simulink model "SPwm_FOC_5phase"  (R2024b)
settings: Solver=VariableStepAuto  StartTime=0.0  StopTime=0.5  RelTol=1e-3
InitFcn:
  | Pn=4;
  | Ts=5e-7;
  | Tsample=1e-4;
  | Ld=1.35e-3;
  | Lq=1.35e-3;
  | R=2.875;
  | flux=0.05;
  | J=0.002;
  | B=0.02;
  | fc=500;
libraries: spsIGBTDiodeLib x10, spsVIMeasurementModel x7, spsCurrentMeasurementLib x5, spsVoltageMeasurementLib x5, slpidlib x5, spsGroundLib x2, spsDCVoltageSourceLib x1, spsPermanentMagnetSynchronousMachineLib x1, sps_lib x1, simulink x1
settings Model: Creator=23954  LastModifiedBy=23954

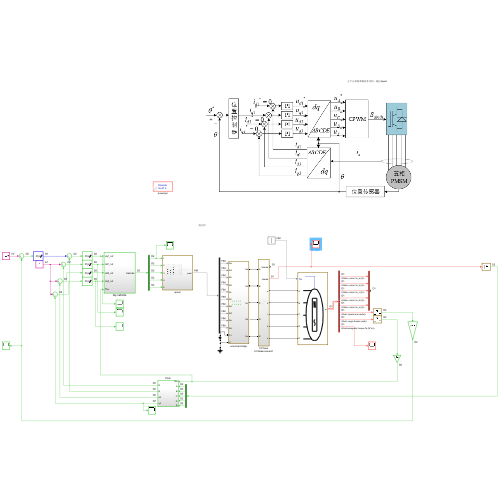
[thumbnail: Simulink's stored preview of the top-level diagram]
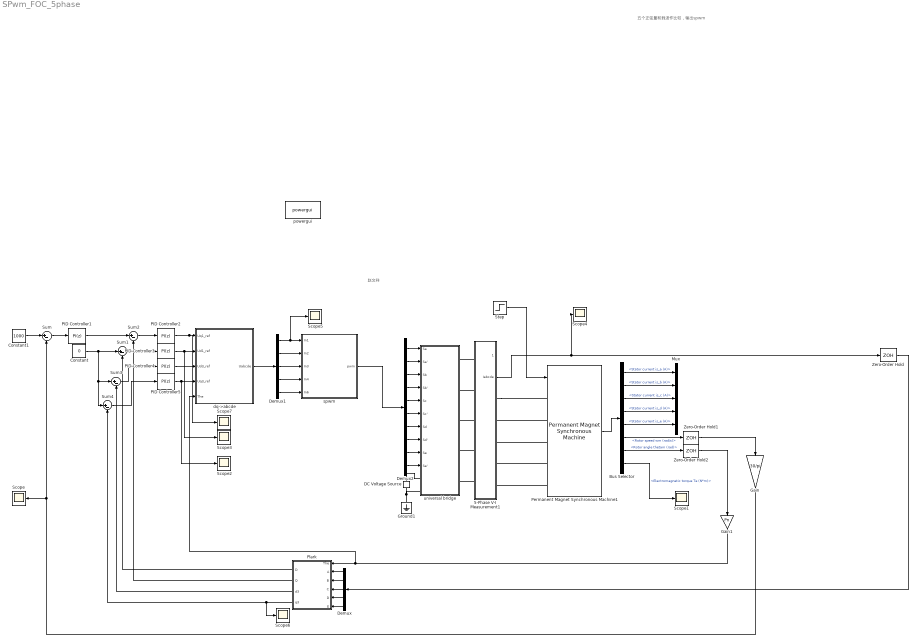
== system SPwm_FOC_5phase ==
  note: 赵文祥
  note: 五个正弦量和载波作比较，输出spwm
  5-Phase V-I Measurement1 : Subsystem
  Bus Selector : BusSelector  OutputSignals=Stator current is_a (A),Stator current is_b (A),Stator current is_c (A),Stator current is_d (A),Stator current is_e (A),Rotor speed wm (rad/s),Rotor angle thetam (rad),Electromagnetic torque Te (N*m)
  Constant : Constant  Value=0
  Constant1 : Constant  Value=1000
  DC Voltage Source : spsDCVoltageSourceLib/DC Voltage Source  Amplitude=311  Measurements=None
  Demux : Demux  Outputs=5
  Demux1 : Demux  Outputs=5
  Demux2 : Demux  Outputs=10
  Gain : Gain  Gain=30/pi
  Gain1 : Gain  Gain=Pn
  Ground1 : spsGroundLib/Ground  LConnTagsString=a
  Mux : Mux  Inputs=5
  PID Controller1 : slpidlib/PID Controller  Controller=PI  Form=Parallel  TimeDomain=Discrete-time  UseExternalTs=off  SampleTime=1e-3  IntegratorMethod=Forward Euler  FilterMethod=Forward Euler  ControllerParametersSource=internal  P=0.02  I=0.02*20  UseKiTs=off  D=0  UseExternalDerivativeSource=off  N=100  UseFilter=on  TunerSelectOption=Transfer Function Based (PID Tuner App)  InitialConditionSource=internal  InitialConditionForIntegrator=0  InitialConditionForFilter=0  DifferentiatorICPrevScaledInput=0  ExternalReset=none  TrackingMode=off  Kt=1  LimitOutput=on  SatLimitsSource=internal  UpperSaturationLimit=150  LowerSaturationLimit=-150  LinearizeAsGain=on  AntiWindupMode=none  Kb=1  LimitIntegrator=off  UpperIntegratorSaturationLimit=inf  LowerIntegratorSaturationLimit=-inf  POutMin=[]  POutMax=[]  IOutMin=[]  IOutMax=[]  DOutMin=[]  DOutMax=[]  NOutMin=[]  NOutMax=[]  SumOutMin=[]  SumOutMax=[]  SaturationOutMin=[]  SaturationOutMax=[]  PParamMin=[]  PParamMax=[]  IParamMin=[]  IParamMax=[]  DParamMin=[]  DParamMax=[]  NParamMin=[]  NParamMax=[]  KbParamMin=[]  KbParamMax=[]  KtParamMin=[]  KtParamMax=[]  KbOutMin=[]  KbOutMax=[]  KtOutMin=[]  KtOutMax=[]  IntegratorOutMin=[]  IntegratorOutMax=[]  FilterOutMin=[]  FilterOutMax=[]  SumI1OutMin=[]  SumI1OutMax=[]  SumI2OutMin=[]  SumI2OutMax=[]  SumI3OutMin=[]  SumI3OutMax=[]  SumI4OutMin=[]  SumI4OutMax=[]  SumDOutMin=[]  SumDOutMax=[]  DifferentiatorOutMin=[]  DifferentiatorOutMax=[]  FilterDiffOutCoefMin=[]  FilterDiffOutCoefMax=[]  ReciprocalOutMin=[]  ReciprocalOutMax=[]  SumDenOutMin=[]  SumDenOutMax=[]  SumNumOutMin=[]  SumNumOutMax=[]  DivideOutMin=[]  DivideOutMax=[]  UdiffTsProdOutMin=[]  UdiffTsProdOutMax=[]  NTsProdOutMin=[]  NTsProdOutMax=[]  UintegralTsProdOutMin=[]  UintegralTsProdOutMax=[]  UngainTsProdOutMin=[]  UngainTsProdOutMax=[]  ClampingZeroOutDataTypeStr=Inherit: Inherit via back propagation  ClampingZeroOutMin=[]  ClampingZeroOutMax=[]  FilterDenConstantOutDataTypeStr=Inherit: Inherit via back propagation  FilterDenConstantOutMin=[]  FilterDenConstantOutMax=[]  PCopyOutDataTypeStr=Inherit: Inherit via back propagation  PCopyOutMin=[]  PCopyOutMax=[]  NCopyOutDataTypeStr=Inherit: Inherit via back propagation  NCopyOutMin=[]  NCopyOutMax=[]  IntegratorContinuousStateAttributes=''  IntegratorStateMustResolveToSignalObject=off  IntegratorRTWStateStorageClass=Auto  FilterContinuousStateAttributes=''  FilterStateMustResolveToSignalObject=off  FilterRTWStateStorageClass=Auto  ParallelPVariant=InternalParameters  IdealPVariant=Disabled  IVariant=InternalParameters  DVariant=Disabled  IntegratorVariant=Discrete  SatVariant=Enabled  AWVariant=Passthrough  PCopyVariant=Disabled  TRVariant=Disabled  FdbkBlocksVariant=Forward  IdealPFdbkVariant=Disabled  SatFdbkVariant=Disabled  DerivativeFilterVariant=Disabled  NVariant=Disabled  NCopyVariant=Disabled_SignalSpec  FilterICVariant=Disabled  IntegratorICVariant=InternalICs  ExternalResetVariant=Disabled  TRSumVariant=Passthrough  SumFdbkVariant=Disabled  SumVariant=Sum_PI  TsampFilterVariant=InternalTs  TsampNgainVariant=Passthrough  TsampIntegralVariant=Disabled_SignalSpec  ExternalSaturationOutDataTypeStr=Inherit: Same as second input  DerivativeSourceVariant=Disabled  PreIntVariant=InternalPreInt
  PID Controller2 : slpidlib/PID Controller  Controller=PI  Form=Parallel  TimeDomain=Discrete-time  UseExternalTs=off  SampleTime=Tsample  IntegratorMethod=Forward Euler  FilterMethod=Forward Euler  ControllerParametersSource=internal  P=Lq*1000  I=R*1100  UseKiTs=off  D=0  UseExternalDerivativeSource=off  N=100  UseFilter=on  TunerSelectOption=Transfer Function Based (PID Tuner App)  InitialConditionSource=internal  InitialConditionForIntegrator=0  InitialConditionForFilter=0  DifferentiatorICPrevScaledInput=0  ExternalReset=none  TrackingMode=off  Kt=1  LimitOutput=on  SatLimitsSource=internal  UpperSaturationLimit=150  LowerSaturationLimit=-150  LinearizeAsGain=on  AntiWindupMode=none  Kb=1  LimitIntegrator=off  UpperIntegratorSaturationLimit=inf  LowerIntegratorSaturationLimit=-inf  POutMin=[]  POutMax=[]  IOutMin=[]  IOutMax=[]  DOutMin=[]  DOutMax=[]  NOutMin=[]  NOutMax=[]  SumOutMin=[]  SumOutMax=[]  SaturationOutMin=[]  SaturationOutMax=[]  PParamMin=[]  PParamMax=[]  IParamMin=[]  IParamMax=[]  DParamMin=[]  DParamMax=[]  NParamMin=[]  NParamMax=[]  KbParamMin=[]  KbParamMax=[]  KtParamMin=[]  KtParamMax=[]  KbOutMin=[]  KbOutMax=[]  KtOutMin=[]  KtOutMax=[]  IntegratorOutMin=[]  IntegratorOutMax=[]  FilterOutMin=[]  FilterOutMax=[]  SumI1OutMin=[]  SumI1OutMax=[]  SumI2OutMin=[]  SumI2OutMax=[]  SumI3OutMin=[]  SumI3OutMax=[]  SumI4OutMin=[]  SumI4OutMax=[]  SumDOutMin=[]  SumDOutMax=[]  DifferentiatorOutMin=[]  DifferentiatorOutMax=[]  FilterDiffOutCoefMin=[]  FilterDiffOutCoefMax=[]  ReciprocalOutMin=[]  ReciprocalOutMax=[]  SumDenOutMin=[]  SumDenOutMax=[]  SumNumOutMin=[]  SumNumOutMax=[]  DivideOutMin=[]  DivideOutMax=[]  UdiffTsProdOutMin=[]  UdiffTsProdOutMax=[]  NTsProdOutMin=[]  NTsProdOutMax=[]  UintegralTsProdOutMin=[]  UintegralTsProdOutMax=[]  UngainTsProdOutMin=[]  UngainTsProdOutMax=[]  ClampingZeroOutDataTypeStr=Inherit: Inherit via back propagation  ClampingZeroOutMin=[]  ClampingZeroOutMax=[]  FilterDenConstantOutDataTypeStr=Inherit: Inherit via back propagation  FilterDenConstantOutMin=[]  FilterDenConstantOutMax=[]  PCopyOutDataTypeStr=Inherit: Inherit via back propagation  PCopyOutMin=[]  PCopyOutMax=[]  NCopyOutDataTypeStr=Inherit: Inherit via back propagation  NCopyOutMin=[]  NCopyOutMax=[]  IntegratorContinuousStateAttributes=''  IntegratorStateMustResolveToSignalObject=off  IntegratorRTWStateStorageClass=Auto  FilterContinuousStateAttributes=''  FilterStateMustResolveToSignalObject=off  FilterRTWStateStorageClass=Auto  ParallelPVariant=InternalParameters  IdealPVariant=Disabled  IVariant=InternalParameters  DVariant=Disabled  IntegratorVariant=Discrete  SatVariant=Enabled  AWVariant=Passthrough  PCopyVariant=Disabled  TRVariant=Disabled  FdbkBlocksVariant=Forward  IdealPFdbkVariant=Disabled  SatFdbkVariant=Disabled  DerivativeFilterVariant=Disabled  NVariant=Disabled  NCopyVariant=Disabled_SignalSpec  FilterICVariant=Disabled  IntegratorICVariant=InternalICs  ExternalResetVariant=Disabled  TRSumVariant=Passthrough  SumFdbkVariant=Disabled  SumVariant=Sum_PI  TsampFilterVariant=InternalTs  TsampNgainVariant=Passthrough  TsampIntegralVariant=Disabled_SignalSpec  ExternalSaturationOutDataTypeStr=Inherit: Same as second input  DerivativeSourceVariant=Disabled  PreIntVariant=InternalPreInt
  PID Controller3 : slpidlib/PID Controller  Controller=PI  Form=Parallel  TimeDomain=Discrete-time  UseExternalTs=off  SampleTime=Tsample  IntegratorMethod=Forward Euler  FilterMethod=Forward Euler  ControllerParametersSource=internal  P=Ld*1000  I=R*1100  UseKiTs=off  D=0  UseExternalDerivativeSource=off  N=100  UseFilter=on  TunerSelectOption=Transfer Function Based (PID Tuner App)  InitialConditionSource=internal  InitialConditionForIntegrator=0  InitialConditionForFilter=0  DifferentiatorICPrevScaledInput=0  ExternalReset=none  TrackingMode=off  Kt=1  LimitOutput=on  SatLimitsSource=internal  UpperSaturationLimit=150  LowerSaturationLimit=-150  LinearizeAsGain=on  AntiWindupMode=none  Kb=1  LimitIntegrator=off  UpperIntegratorSaturationLimit=inf  LowerIntegratorSaturationLimit=-inf  POutMin=[]  POutMax=[]  IOutMin=[]  IOutMax=[]  DOutMin=[]  DOutMax=[]  NOutMin=[]  NOutMax=[]  SumOutMin=[]  SumOutMax=[]  SaturationOutMin=[]  SaturationOutMax=[]  PParamMin=[]  PParamMax=[]  IParamMin=[]  IParamMax=[]  DParamMin=[]  DParamMax=[]  NParamMin=[]  NParamMax=[]  KbParamMin=[]  KbParamMax=[]  KtParamMin=[]  KtParamMax=[]  KbOutMin=[]  KbOutMax=[]  KtOutMin=[]  KtOutMax=[]  IntegratorOutMin=[]  IntegratorOutMax=[]  FilterOutMin=[]  FilterOutMax=[]  SumI1OutMin=[]  SumI1OutMax=[]  SumI2OutMin=[]  SumI2OutMax=[]  SumI3OutMin=[]  SumI3OutMax=[]  SumI4OutMin=[]  SumI4OutMax=[]  SumDOutMin=[]  SumDOutMax=[]  DifferentiatorOutMin=[]  DifferentiatorOutMax=[]  FilterDiffOutCoefMin=[]  FilterDiffOutCoefMax=[]  ReciprocalOutMin=[]  ReciprocalOutMax=[]  SumDenOutMin=[]  SumDenOutMax=[]  SumNumOutMin=[]  SumNumOutMax=[]  DivideOutMin=[]  DivideOutMax=[]  UdiffTsProdOutMin=[]  UdiffTsProdOutMax=[]  NTsProdOutMin=[]  NTsProdOutMax=[]  UintegralTsProdOutMin=[]  UintegralTsProdOutMax=[]  UngainTsProdOutMin=[]  UngainTsProdOutMax=[]  ClampingZeroOutDataTypeStr=Inherit: Inherit via back propagation  ClampingZeroOutMin=[]  ClampingZeroOutMax=[]  FilterDenConstantOutDataTypeStr=Inherit: Inherit via back propagation  FilterDenConstantOutMin=[]  FilterDenConstantOutMax=[]  PCopyOutDataTypeStr=Inherit: Inherit via back propagation  PCopyOutMin=[]  PCopyOutMax=[]  NCopyOutDataTypeStr=Inherit: Inherit via back propagation  NCopyOutMin=[]  NCopyOutMax=[]  IntegratorContinuousStateAttributes=''  IntegratorStateMustResolveToSignalObject=off  IntegratorRTWStateStorageClass=Auto  FilterContinuousStateAttributes=''  FilterStateMustResolveToSignalObject=off  FilterRTWStateStorageClass=Auto  ParallelPVariant=InternalParameters  IdealPVariant=Disabled  IVariant=InternalParameters  DVariant=Disabled  IntegratorVariant=Discrete  SatVariant=Enabled  AWVariant=Passthrough  PCopyVariant=Disabled  TRVariant=Disabled  FdbkBlocksVariant=Forward  IdealPFdbkVariant=Disabled  SatFdbkVariant=Disabled  DerivativeFilterVariant=Disabled  NVariant=Disabled  NCopyVariant=Disabled_SignalSpec  FilterICVariant=Disabled  IntegratorICVariant=InternalICs  ExternalResetVariant=Disabled  TRSumVariant=Passthrough  SumFdbkVariant=Disabled  SumVariant=Sum_PI  TsampFilterVariant=InternalTs  TsampNgainVariant=Passthrough  TsampIntegralVariant=Disabled_SignalSpec  ExternalSaturationOutDataTypeStr=Inherit: Same as second input  DerivativeSourceVariant=Disabled  PreIntVariant=InternalPreInt
  PID Controller4 : slpidlib/PID Controller  Controller=PI  Form=Parallel  TimeDomain=Discrete-time  UseExternalTs=off  SampleTime=Tsample  IntegratorMethod=Forward Euler  FilterMethod=Forward Euler  ControllerParametersSource=internal  P=Ld*1000  I=R*1100  UseKiTs=off  D=0  UseExternalDerivativeSource=off  N=100  UseFilter=on  TunerSelectOption=Transfer Function Based (PID Tuner App)  InitialConditionSource=internal  InitialConditionForIntegrator=0  InitialConditionForFilter=0  DifferentiatorICPrevScaledInput=0  ExternalReset=none  TrackingMode=off  Kt=1  LimitOutput=on  SatLimitsSource=internal  UpperSaturationLimit=150  LowerSaturationLimit=-150  LinearizeAsGain=on  AntiWindupMode=none  Kb=1  LimitIntegrator=off  UpperIntegratorSaturationLimit=inf  LowerIntegratorSaturationLimit=-inf  POutMin=[]  POutMax=[]  IOutMin=[]  IOutMax=[]  DOutMin=[]  DOutMax=[]  NOutMin=[]  NOutMax=[]  SumOutMin=[]  SumOutMax=[]  SaturationOutMin=[]  SaturationOutMax=[]  PParamMin=[]  PParamMax=[]  IParamMin=[]  IParamMax=[]  DParamMin=[]  DParamMax=[]  NParamMin=[]  NParamMax=[]  KbParamMin=[]  KbParamMax=[]  KtParamMin=[]  KtParamMax=[]  KbOutMin=[]  KbOutMax=[]  KtOutMin=[]  KtOutMax=[]  IntegratorOutMin=[]  IntegratorOutMax=[]  FilterOutMin=[]  FilterOutMax=[]  SumI1OutMin=[]  SumI1OutMax=[]  SumI2OutMin=[]  SumI2OutMax=[]  SumI3OutMin=[]  SumI3OutMax=[]  SumI4OutMin=[]  SumI4OutMax=[]  SumDOutMin=[]  SumDOutMax=[]  DifferentiatorOutMin=[]  DifferentiatorOutMax=[]  FilterDiffOutCoefMin=[]  FilterDiffOutCoefMax=[]  ReciprocalOutMin=[]  ReciprocalOutMax=[]  SumDenOutMin=[]  SumDenOutMax=[]  SumNumOutMin=[]  SumNumOutMax=[]  DivideOutMin=[]  DivideOutMax=[]  UdiffTsProdOutMin=[]  UdiffTsProdOutMax=[]  NTsProdOutMin=[]  NTsProdOutMax=[]  UintegralTsProdOutMin=[]  UintegralTsProdOutMax=[]  UngainTsProdOutMin=[]  UngainTsProdOutMax=[]  ClampingZeroOutDataTypeStr=Inherit: Inherit via back propagation  ClampingZeroOutMin=[]  ClampingZeroOutMax=[]  FilterDenConstantOutDataTypeStr=Inherit: Inherit via back propagation  FilterDenConstantOutMin=[]  FilterDenConstantOutMax=[]  PCopyOutDataTypeStr=Inherit: Inherit via back propagation  PCopyOutMin=[]  PCopyOutMax=[]  NCopyOutDataTypeStr=Inherit: Inherit via back propagation  NCopyOutMin=[]  NCopyOutMax=[]  IntegratorContinuousStateAttributes=''  IntegratorStateMustResolveToSignalObject=off  IntegratorRTWStateStorageClass=Auto  FilterContinuousStateAttributes=''  FilterStateMustResolveToSignalObject=off  FilterRTWStateStorageClass=Auto  ParallelPVariant=InternalParameters  IdealPVariant=Disabled  IVariant=InternalParameters  DVariant=Disabled  IntegratorVariant=Discrete  SatVariant=Enabled  AWVariant=Passthrough  PCopyVariant=Disabled  TRVariant=Disabled  FdbkBlocksVariant=Forward  IdealPFdbkVariant=Disabled  SatFdbkVariant=Disabled  DerivativeFilterVariant=Disabled  NVariant=Disabled  NCopyVariant=Disabled_SignalSpec  FilterICVariant=Disabled  IntegratorICVariant=InternalICs  ExternalResetVariant=Disabled  TRSumVariant=Passthrough  SumFdbkVariant=Disabled  SumVariant=Sum_PI  TsampFilterVariant=InternalTs  TsampNgainVariant=Passthrough  TsampIntegralVariant=Disabled_SignalSpec  ExternalSaturationOutDataTypeStr=Inherit: Same as second input  DerivativeSourceVariant=Disabled  PreIntVariant=InternalPreInt
  PID Controller5 : slpidlib/PID Controller  Controller=PI  Form=Parallel  TimeDomain=Discrete-time  UseExternalTs=off  SampleTime=Tsample  IntegratorMethod=Forward Euler  FilterMethod=Forward Euler  ControllerParametersSource=internal  P=Lq*1000  I=R*1100  UseKiTs=off  D=0  UseExternalDerivativeSource=off  N=100  UseFilter=on  TunerSelectOption=Transfer Function Based (PID Tuner App)  InitialConditionSource=internal  InitialConditionForIntegrator=0  InitialConditionForFilter=0  DifferentiatorICPrevScaledInput=0  ExternalReset=none  TrackingMode=off  Kt=1  LimitOutput=on  SatLimitsSource=internal  UpperSaturationLimit=150  LowerSaturationLimit=-150  LinearizeAsGain=on  AntiWindupMode=none  Kb=1  LimitIntegrator=off  UpperIntegratorSaturationLimit=inf  LowerIntegratorSaturationLimit=-inf  POutMin=[]  POutMax=[]  IOutMin=[]  IOutMax=[]  DOutMin=[]  DOutMax=[]  NOutMin=[]  NOutMax=[]  SumOutMin=[]  SumOutMax=[]  SaturationOutMin=[]  SaturationOutMax=[]  PParamMin=[]  PParamMax=[]  IParamMin=[]  IParamMax=[]  DParamMin=[]  DParamMax=[]  NParamMin=[]  NParamMax=[]  KbParamMin=[]  KbParamMax=[]  KtParamMin=[]  KtParamMax=[]  KbOutMin=[]  KbOutMax=[]  KtOutMin=[]  KtOutMax=[]  IntegratorOutMin=[]  IntegratorOutMax=[]  FilterOutMin=[]  FilterOutMax=[]  SumI1OutMin=[]  SumI1OutMax=[]  SumI2OutMin=[]  SumI2OutMax=[]  SumI3OutMin=[]  SumI3OutMax=[]  SumI4OutMin=[]  SumI4OutMax=[]  SumDOutMin=[]  SumDOutMax=[]  DifferentiatorOutMin=[]  DifferentiatorOutMax=[]  FilterDiffOutCoefMin=[]  FilterDiffOutCoefMax=[]  ReciprocalOutMin=[]  ReciprocalOutMax=[]  SumDenOutMin=[]  SumDenOutMax=[]  SumNumOutMin=[]  SumNumOutMax=[]  DivideOutMin=[]  DivideOutMax=[]  UdiffTsProdOutMin=[]  UdiffTsProdOutMax=[]  NTsProdOutMin=[]  NTsProdOutMax=[]  UintegralTsProdOutMin=[]  UintegralTsProdOutMax=[]  UngainTsProdOutMin=[]  UngainTsProdOutMax=[]  ClampingZeroOutDataTypeStr=Inherit: Inherit via back propagation  ClampingZeroOutMin=[]  ClampingZeroOutMax=[]  FilterDenConstantOutDataTypeStr=Inherit: Inherit via back propagation  FilterDenConstantOutMin=[]  FilterDenConstantOutMax=[]  PCopyOutDataTypeStr=Inherit: Inherit via back propagation  PCopyOutMin=[]  PCopyOutMax=[]  NCopyOutDataTypeStr=Inherit: Inherit via back propagation  NCopyOutMin=[]  NCopyOutMax=[]  IntegratorContinuousStateAttributes=''  IntegratorStateMustResolveToSignalObject=off  IntegratorRTWStateStorageClass=Auto  FilterContinuousStateAttributes=''  FilterStateMustResolveToSignalObject=off  FilterRTWStateStorageClass=Auto  ParallelPVariant=InternalParameters  IdealPVariant=Disabled  IVariant=InternalParameters  DVariant=Disabled  IntegratorVariant=Discrete  SatVariant=Enabled  AWVariant=Passthrough  PCopyVariant=Disabled  TRVariant=Disabled  FdbkBlocksVariant=Forward  IdealPFdbkVariant=Disabled  SatFdbkVariant=Disabled  DerivativeFilterVariant=Disabled  NVariant=Disabled  NCopyVariant=Disabled_SignalSpec  FilterICVariant=Disabled  IntegratorICVariant=InternalICs  ExternalResetVariant=Disabled  TRSumVariant=Passthrough  SumFdbkVariant=Disabled  SumVariant=Sum_PI  TsampFilterVariant=InternalTs  TsampNgainVariant=Passthrough  TsampIntegralVariant=Disabled_SignalSpec  ExternalSaturationOutDataTypeStr=Inherit: Same as second input  DerivativeSourceVariant=Disabled  PreIntVariant=InternalPreInt
  Permanent Magnet Synchronous Machine1 : spsPermanentMagnetSynchronousMachineLib/Permanent Magnet Synchronous Machine  NbPhases=5  FluxDistribution=Sinusoidal  RotorType=Round  MechanicalLoad=Torque Tm  PresetModel=No  ShowDetailedParameters=on  MeasurementBus=off  Resistance=R  Inductance=8.5e-3  dqInductances=[8.5e-3,8.5e-3]  La=Ld  MachineConstant=Flux linkage established by magnets (V.s)  Flux=flux  VoltageCst=24.6211  TorqueCst=0.5  Flat=120  Mechanical=[J B Pn 0]  PolePairs=4  InitialConditions=[0,0, 0,0]  InitialConditions5ph=[0 0 0 0 0 0]  RefAngle=Aligned with phase A axis (original Park)  IterativeDiscreteModel=Trapezoidal non iterative  TsBlock=-1  TsPowergui=0
  Plark : Subsystem
  Scope{,1..7} (8 alike) : Scope
  Step : Step  Time=0.35  After=0  SampleTime=0
  Sum{,1..4} (5 alike) : Sum  Inputs=|+-
  Zero-Order Hold : ZeroOrderHold  SampleTime=1e-4
  Zero-Order Hold1 : ZeroOrderHold  SampleTime=1e-4
  Zero-Order Hold2 : ZeroOrderHold  SampleTime=1e-4
  dq->abcde : Subsystem
  powergui : sps_lib/powergui  Priority=1  SimulationMode=Discrete  SampleTime=Ts  frequency=60  Iterations=50  frequencyindice=0  Pbase=100e6  ErrMax=1e-4  UnitsV=kV  UnitsW=MW  buscounter=0  FunctionMessages=off  echomessages=off  EnableUseOfTLC=off  CurrentSourceSwitches=off  DisableSnubberDevices=off  DisableRonSwitches=off  DisableVfSwitches=off  DisplayEquations=off  AutomaticDiscreteSolvers=off  SolverType=Tustin/Backward Euler (TBE)  Interpol=off  ExternalGateDelay=off  methode=off  Ts=100  x0status=blocks  SPID=on  SwTol=0  HookPort=off  NonlinearTolerance=1e-4  nMaxIteration=100  ContinueOnMaxIteration=off  RestoreLinks=warning  ResistiveCurrentMeasurement=off  Frange=[0:2:500]  Ylog=off  Xlog=on  ShowGrid=off  save=off  variable=ZData  structure=0  ZoomFFT=off  StartTime=0.0  cycles=1  DisplayStyle=1  fundamental=60  FreqAxis=off  MaxFrequency=1000  frequencyindicesteady=1  RmsSteady=1  display=off
  spwm : Subsystem
  universal bridge : Subsystem
  wires:
  Gain/1 -> Sum/2, Scope/1
  Bus Selector/4 -> Mux/4  "<Stator current is_d (A)>"
  PID Controller1/1 -> Sum2/1
  Bus Selector/2 -> Mux/2  "<Stator current is_b (A)>"
  Zero-Order Hold2/1 -> Gain1/1
  Bus Selector/5 -> Mux/5  "<Stator current is_e (A)>"
  Permanent Magnet Synchronous Machine1/1 -> Bus Selector/1
  Bus Selector/6 -> Zero-Order Hold1/1  "<Rotor speed wm (rad/s)>"
  Sum/1 -> PID Controller1/1
  Bus Selector/7 -> Zero-Order Hold2/1  "<Rotor angle thetam (rad)>"
  Bus Selector/1 -> Mux/1  "<Stator current is_a (A)>"
  5-Phase V-I Measurement1/2(Iabcde) -> Scope4/1, Zero-Order Hold/1
  Zero-Order Hold1/1 -> Gain/1
  Zero-Order Hold/1 -> Demux/1
  Bus Selector/3 -> Mux/3  "<Stator current is_c (A)>"
  Constant/1 -> Sum4/1, Sum3/1, Sum1/1
  Gain1/1 -> dq->abcde/5(The), Plark/1(The)
  Demux/5 -> Plark/6(E)
  Demux/4 -> Plark/5(D)
  Demux/3 -> Plark/4(C)
  Demux/2 -> Plark/3(B)
  Demux/1 -> Plark/2(A)
  Plark/2(Q) -> Sum2/2
  Plark/1("D ") -> Sum1/2
  Plark/3(d3) -> Sum3/2
  Plark/4(q3) -> Scope6/1, Sum4/2
  dq->abcde/1(Uabcde) -> Demux1/1
  Demux1/4 -> spwm/4(In4)
  Demux1/3 -> spwm/3(In3)
  Demux1/2 -> spwm/2(In2)
  Demux1/1 -> Scope5/1, spwm/1(In1)
  Sum2/1 -> PID Controller2/1
  Sum1/1 -> PID Controller3/1
  Sum3/1 -> PID Controller4/1
  Sum4/1 -> PID Controller5/1
  Demux2/1 -> universal bridge/1(Sa)
  Demux2/2 -> universal bridge/2(Sa')
  Demux2/3 -> universal bridge/3(Sb)
  Demux2/4 -> universal bridge/4(Sb')
  Demux2/5 -> universal bridge/5(Sc)
  Demux2/6 -> universal bridge/6(Sc')
  Demux2/7 -> universal bridge/7(Sd)
  Demux2/8 -> universal bridge/8(Sd')
  Demux2/9 -> universal bridge/9(Se)
  Demux2/10 -> universal bridge/10(Se')
  PID Controller2/1 -> Scope7/1, dq->abcde/1("Uq1_ref ")
  PID Controller3/1 -> dq->abcde/2(Ud1_ref), Scope3/1
  PID Controller5/1 -> Scope2/1, dq->abcde/4(Uq3_ref)
  PID Controller4/1 -> dq->abcde/3(Ud3_ref)
  Bus Selector/8 -> Scope1/1  "<Electromagnetic torque Te (N*m)>"
  Step/1 -> Permanent Magnet Synchronous Machine1/1
  Demux1/5 -> spwm/5(In6)
  spwm/1(pwm) -> Demux2/1
  Constant1/1 -> Sum/1
  connections:
  DC Voltage Source/RConn1 -- universal bridge/LConn1
  DC Voltage Source/LConn1 -- universal bridge/LConn2 -- Ground1/LConn1
  5-Phase V-I Measurement1/LConn1 -- universal bridge/RConn1
  5-Phase V-I Measurement1/LConn2 -- universal bridge/RConn2
  5-Phase V-I Measurement1/LConn3 -- universal bridge/RConn3
  5-Phase V-I Measurement1/LConn4 -- universal bridge/RConn4
  5-Phase V-I Measurement1/LConn5 -- universal bridge/RConn5
  5-Phase V-I Measurement1/RConn1 -- Permanent Magnet Synchronous Machine1/LConn1
  Permanent Magnet Synchronous Machine1/LConn5 -- 5-Phase V-I Measurement1/RConn5
  Permanent Magnet Synchronous Machine1/LConn4 -- 5-Phase V-I Measurement1/RConn4
  Permanent Magnet Synchronous Machine1/LConn3 -- 5-Phase V-I Measurement1/RConn3
  Permanent Magnet Synchronous Machine1/LConn2 -- 5-Phase V-I Measurement1/RConn2

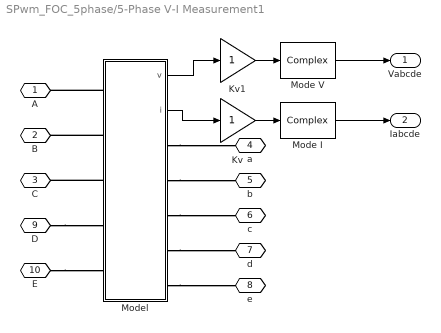
== system SPwm_FOC_5phase/5-Phase V-I Measurement1 ==
  Kv : Gain  SaturateOnIntegerOverflow=on  OutDataTypeStr=Inherit: Same as input  ParamDataTypeStr=Inherit: Same as input
  Kv1 : Gain  SaturateOnIntegerOverflow=on  OutDataTypeStr=Inherit: Same as input  ParamDataTypeStr=Inherit: Same as input
  Mode I : spsVIMeasurementModel/Complex  SystemSampleTime=-1  VariantActivationTime=update diagram  AllowFlexibleInterface=on  Latency=0  AutoFrameSizeCalculation=off
  Mode V : spsVIMeasurementModel/Complex  SystemSampleTime=-1  VariantActivationTime=update diagram  AllowFlexibleInterface=on  Latency=0  AutoFrameSizeCalculation=off
  Model : Subsystem  mask(Specialized Power Systems Three-Phase VI Measurement){}
  A : PMIOPort  Side=Left
  B : PMIOPort  Port=2  Side=Left
  C : PMIOPort  Port=3  Side=Left
  a : PMIOPort  Port=4  Side=Right
  b : PMIOPort  Port=5  Side=Right
  c : PMIOPort  Port=6  Side=Right
  d : PMIOPort  Port=7  Side=Right
  e : PMIOPort  Port=8  Side=Right
  D : PMIOPort  Port=9  Side=Left
  E : PMIOPort  Port=10  Side=Left
  Vabcde : Outport  VectorParamsAs1DForOutWhenUnconnected=off
  Iabcde : Outport  Port=2  VectorParamsAs1DForOutWhenUnconnected=off
  wires:
  Mode V/1 -> Vabcde/1
  Model/2(i) -> Kv/1
  Mode I/1 -> Iabcde/1
  Kv/1 -> Mode I/1
  Model/1(v) -> Kv1/1
  Kv1/1 -> Mode V/1
  connections:
  Model/RConn5 -- e/RConn1
  Model/RConn4 -- d/RConn1
  E/RConn1 -- Model/LConn5
  D/RConn1 -- Model/LConn4
  Model/LConn3 -- C/RConn1
  Model/LConn1 -- A/RConn1
  Model/RConn1 -- a/RConn1
  Model/RConn2 -- b/RConn1
  Model/LConn2 -- B/RConn1
  Model/RConn3 -- c/RConn1

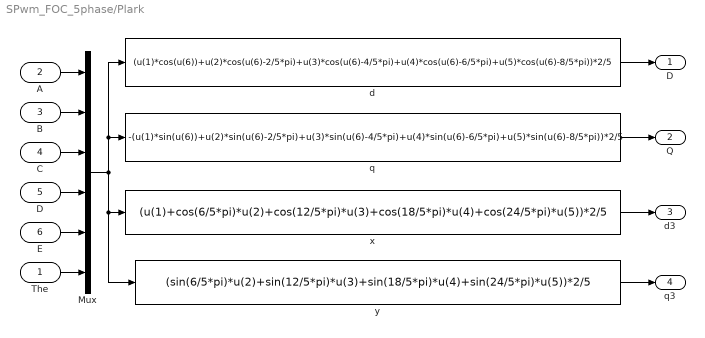
== system SPwm_FOC_5phase/Plark ==
  The : Inport
  A : Inport  Port=2
  B : Inport  Port=3
  C : Inport  Port=4
  D : Inport  Port=5
  E : Inport  Port=6
  Mux : Mux  Inputs=6
  d : Fcn  Expr=(u(1)*cos(u(6))+u(2)*cos(u(6)-2/5*pi)+u(3)*cos(u(6)-4/5*pi)+u(4)*cos(u(6)-6/5*pi)+u(5)*cos(u(6)-8/5*pi))*2/5
  q : Fcn  Expr=-(u(1)*sin(u(6))+u(2)*sin(u(6)-2/5*pi)+u(3)*sin(u(6)-4/5*pi)+u(4)*sin(u(6)-6/5*pi)+u(5)*sin(u(6)-8/5*pi))*2/5
  "x " : Fcn  Expr=(u(1)+cos(6/5*pi)*u(2)+cos(12/5*pi)*u(3)+cos(18/5*pi)*u(4)+cos(24/5*pi)*u(5))*2/5
  "y " : Fcn  Expr=(sin(6/5*pi)*u(2)+sin(12/5*pi)*u(3)+sin(18/5*pi)*u(4)+sin(24/5*pi)*u(5))*2/5
  "D " : Outport
  Q : Outport  Port=2
  d3 : Outport  Port=3
  q3 : Outport  Port=4
  wires:
  "y "/1 -> q3/1
  "x "/1 -> d3/1
  q/1 -> Q/1
  Mux/1 -> "x "/1, "y "/1, d/1, q/1
  The/1 -> Mux/6
  E/1 -> Mux/5
  D/1 -> Mux/4
  A/1 -> Mux/1
  C/1 -> Mux/3
  B/1 -> Mux/2
  d/1 -> "D "/1

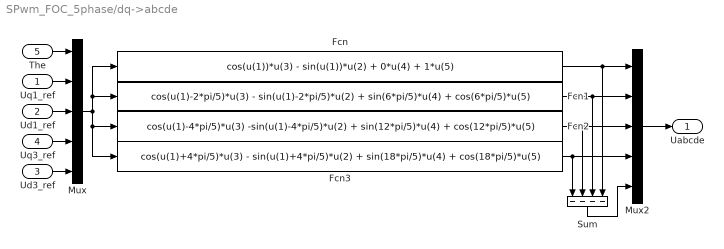
== system SPwm_FOC_5phase/dq->abcde ==
  "Uq1_ref " : Inport
  Ud1_ref : Inport  Port=2
  Ud3_ref : Inport  Port=3
  Uq3_ref : Inport  Port=4
  The : Inport  Port=5
  Fcn : Fcn  Expr=cos(u(1))*u(3) - sin(u(1))*u(2) + 0*u(4) + 1*u(5)
  Fcn1 : Fcn  Expr=cos(u(1)-2*pi/5)*u(3) - sin(u(1)-2*pi/5)*u(2) + sin(6*pi/5)*u(4) + cos(6*pi/5)*u(5)
  Fcn2 : Fcn  Expr=cos(u(1)-4*pi/5)*u(3) -sin(u(1)-4*pi/5)*u(2) + sin(12*pi/5)*u(4) + cos(12*pi/5)*u(5)
  Fcn3 : Fcn  Expr=cos(u(1)+4*pi/5)*u(3) - sin(u(1)+4*pi/5)*u(2) + sin(18*pi/5)*u(4) + cos(18*pi/5)*u(5)
  Mux : Mux  Inputs=5
  Mux2 : Mux  Inputs=5
  Sum : Sum  Inputs=----  InputSameDT=on  SaturateOnIntegerOverflow=on  OutDataTypeStr=Inherit: Same as first input
  Uabcde : Outport  InitialOutput=0
  wires:
  Sum/1 -> Mux2/5
  Fcn1/1 -> Mux2/2, Sum/3
  Fcn2/1 -> Mux2/3, Sum/2
  Fcn3/1 -> Mux2/4, Sum/1
  Mux/1 -> Fcn2/1, Fcn3/1, Fcn/1, Fcn1/1
  Fcn/1 -> Sum/4, Mux2/1
  The/1 -> Mux/1
  "Uq1_ref "/1 -> Mux/2
  Ud1_ref/1 -> Mux/3
  Uq3_ref/1 -> Mux/4
  Ud3_ref/1 -> Mux/5
  Mux2/1 -> Uabcde/1

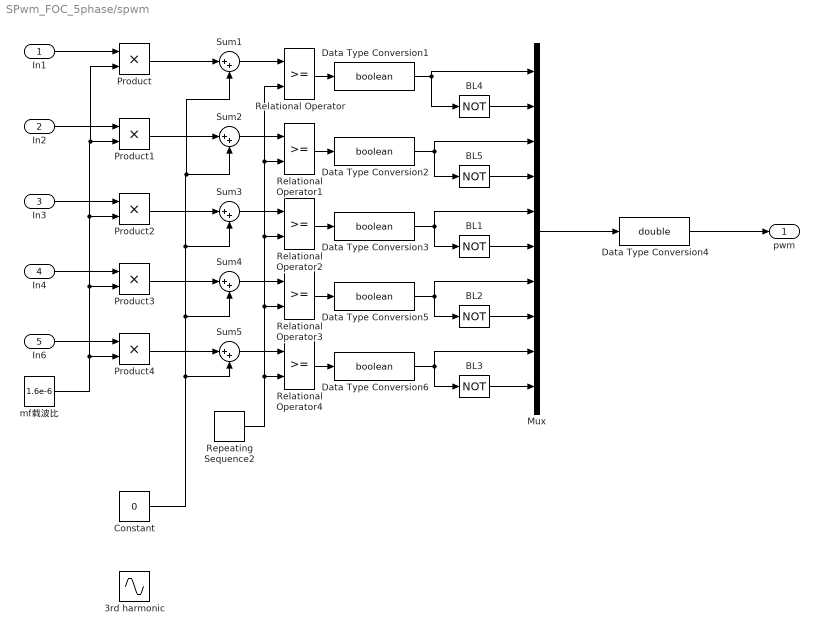
== system SPwm_FOC_5phase/spwm ==
  In1 : Inport
  In2 : Inport  Port=2
  In3 : Inport  Port=3
  In4 : Inport  Port=4
  In6 : Inport  Port=5
  3rd harmonic : Sin  Amplitude=(1/6)*0.7*1.1548  Frequency=6*pi*50  SampleTime=0
  BL{1..5} (5 alike) : Logic  Operator=NOT  Inputs=1
  Constant : Constant  Value=0
  Data Type Conversion{1..3,5..6} (5 alike) : DataTypeConversion  OutDataTypeStr=boolean
  Data Type Conversion4 : DataTypeConversion  OutDataTypeStr=double
  Mux : Mux  Inputs=10
  Product{,1..4} (5 alike) : Product
  Relational Operator{,1..4} (5 alike) : RelationalOperator
  Repeating Sequence2 : simulink/Sources/Repeating Sequence  rep_seq_t=[0 5/10000 1/1000]  rep_seq_y=[0 5/10000 0]
  Sum{1..5} (5 alike) : Sum  Inputs=|++
  mf载波比 : Constant  Value=1.6e-6
  pwm : Outport
  wires:
  Relational Operator2/1 -> Data Type Conversion3/1
  Sum1/1 -> Relational Operator/1
  Product1/1 -> Sum2/1
  Sum2/1 -> Relational Operator1/1
  BL1/1 -> Mux/6
  Product2/1 -> Sum3/1
  Product/1 -> Sum1/1
  Relational Operator1/1 -> Data Type Conversion2/1
  Data Type Conversion2/1 -> Mux/3, BL5/1
  Data Type Conversion1/1 -> BL4/1, Mux/1
  Sum3/1 -> Relational Operator2/1
  BL4/1 -> Mux/2
  Data Type Conversion4/1 -> pwm/1
  BL5/1 -> Mux/4
  Relational Operator/1 -> Data Type Conversion1/1
  Data Type Conversion3/1 -> BL1/1, Mux/5
  Mux/1 -> Data Type Conversion4/1
  In1/1 -> Product/1
  In2/1 -> Product1/1
  In3/1 -> Product2/1
  Data Type Conversion5/1 -> Mux/7, BL2/1
  Product3/1 -> Sum4/1
  BL2/1 -> Mux/8
  Relational Operator3/1 -> Data Type Conversion5/1
  Sum4/1 -> Relational Operator3/1
  Data Type Conversion6/1 -> Mux/9, BL3/1
  Product4/1 -> Sum5/1
  BL3/1 -> Mux/10
  Relational Operator4/1 -> Data Type Conversion6/1
  Sum5/1 -> Relational Operator4/1
  In6/1 -> Product4/1
  In4/1 -> Product3/1
  mf载波比/1 -> Product/2, Product1/2, Product2/2, Product3/2, Product4/2
  Constant/1 -> Sum1/2, Sum2/2, Sum3/2, Sum4/2, Sum5/2
  Repeating Sequence2/1 -> Relational Operator/2, Relational Operator1/2, Relational Operator2/2, Relational Operator3/2, Relational Operator4/2

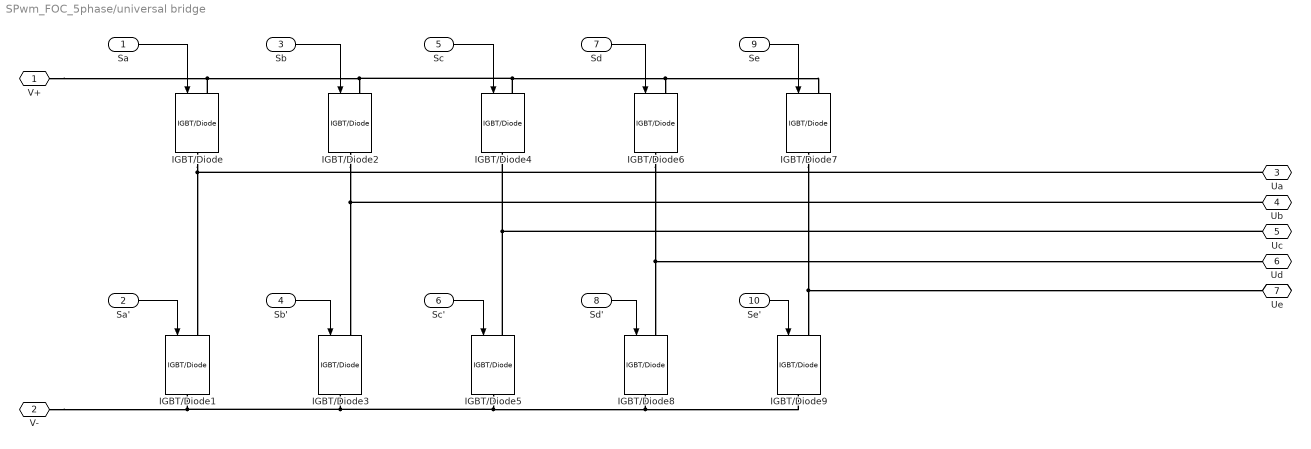
== system SPwm_FOC_5phase/universal bridge ==
  Sa : Inport
  Sa' : Inport  Port=2
  Sb : Inport  Port=3
  Sb' : Inport  Port=4
  Sc : Inport  Port=5
  Sc' : Inport  Port=6
  Sd : Inport  Port=7
  Sd' : Inport  Port=8
  Se : Inport  Port=9
  Se' : Inport  Port=10
  IGBT/Diode{,1..9} (10 alike) : spsIGBTDiodeLib/IGBT//Diode  Ron=1e-3  Rs=1e5  Cs=inf  Measurements=off
  V+ : PMIOPort  Side=Left
  V- : PMIOPort  Port=2  Side=Left
  Ua : PMIOPort  Port=3  Side=Right
  Ub : PMIOPort  Port=4  Side=Right
  Uc : PMIOPort  Port=5  Side=Right
  Ud : PMIOPort  Port=6  Side=Right
  Ue : PMIOPort  Port=7  Side=Right
  wires:
  Sa/1 -> IGBT/Diode/1
  Sb/1 -> IGBT/Diode2/1
  Sb'/1 -> IGBT/Diode3/1
  Sa'/1 -> IGBT/Diode1/1
  Sc'/1 -> IGBT/Diode5/1
  Sc/1 -> IGBT/Diode4/1
  Sd/1 -> IGBT/Diode6/1
  Se/1 -> IGBT/Diode7/1
  Sd'/1 -> IGBT/Diode8/1
  Se'/1 -> IGBT/Diode9/1
  connections:
  IGBT/Diode2/RConn1 -- Ub/RConn1 -- IGBT/Diode3/LConn1
  IGBT/Diode2/LConn1 -- IGBT/Diode7/LConn1 -- IGBT/Diode6/LConn1 -- IGBT/Diode4/LConn1 -- V+/RConn1 -- IGBT/Diode/LConn1
  IGBT/Diode5/RConn1 -- IGBT/Diode9/RConn1 -- IGBT/Diode8/RConn1 -- IGBT/Diode3/RConn1 -- V-/RConn1 -- IGBT/Diode1/RConn1
  IGBT/Diode5/LConn1 -- IGBT/Diode4/RConn1 -- Uc/RConn1
  IGBT/Diode/RConn1 -- IGBT/Diode1/LConn1 -- Ua/RConn1
  IGBT/Diode6/RConn1 -- IGBT/Diode8/LConn1 -- Ud/RConn1
  IGBT/Diode7/RConn1 -- Ue/RConn1 -- IGBT/Diode9/LConn1

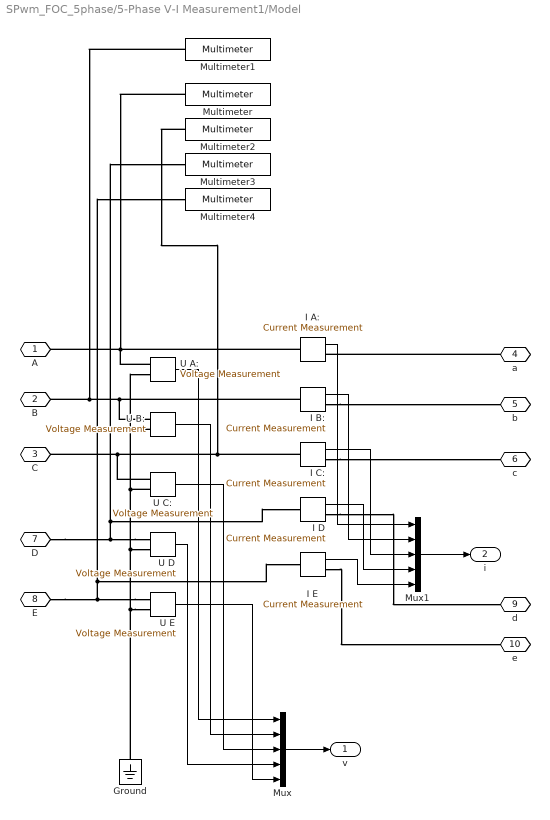
== system SPwm_FOC_5phase/5-Phase V-I Measurement1/Model ==
  Ground : spsGroundLib/Ground  LConnTagsString=a
  I A: : spsCurrentMeasurementLib/Current Measurement  PhasorSimulation=off  OutputType=Complex  PSBequivalent=0
  I B: : spsCurrentMeasurementLib/Current Measurement  PhasorSimulation=off  OutputType=Complex  PSBequivalent=0
  I C: : spsCurrentMeasurementLib/Current Measurement  PhasorSimulation=off  OutputType=Complex  PSBequivalent=0
  I D : spsCurrentMeasurementLib/Current Measurement  PhasorSimulation=off  OutputType=Complex  PSBequivalent=0
  I E : spsCurrentMeasurementLib/Current Measurement  PhasorSimulation=off  OutputType=Complex  PSBequivalent=0
  Multimeter{,1..4} (5 alike) : spsVIMeasurementModel/NO/Multimeter  PhysicalDomain=powersysdomain  SubClassName=unknown  LeftPortType=p1  RightPortType=p1  LConnTagsString=a  RConnTagsString=__new0
  Mux : Mux  Inputs=5
  Mux1 : Mux  Inputs=5
  U A: : spsVoltageMeasurementLib/Voltage Measurement  PhasorSimulation=off  OutputType=Complex  PSBequivalent=0
  U B: : spsVoltageMeasurementLib/Voltage Measurement  PhasorSimulation=off  OutputType=Complex  PSBequivalent=0
  U C: : spsVoltageMeasurementLib/Voltage Measurement  PhasorSimulation=off  OutputType=Complex  PSBequivalent=0
  U D : spsVoltageMeasurementLib/Voltage Measurement  PhasorSimulation=off  OutputType=Complex  PSBequivalent=0
  U E : spsVoltageMeasurementLib/Voltage Measurement  PhasorSimulation=off  OutputType=Complex  PSBequivalent=0
  A : PMIOPort  Side=Left
  B : PMIOPort  Port=2  Side=Left
  C : PMIOPort  Port=3  Side=Left
  a : PMIOPort  Port=4  Side=Right
  b : PMIOPort  Port=5  Side=Right
  c : PMIOPort  Port=6  Side=Right
  D : PMIOPort  Port=7  Side=Left
  E : PMIOPort  Port=8  Side=Left
  d : PMIOPort  Port=9  Side=Right
  e : PMIOPort  Port=10  Side=Right
  v : Outport  VectorParamsAs1DForOutWhenUnconnected=off
  i : Outport  Port=2  VectorParamsAs1DForOutWhenUnconnected=off
  wires:
  I E/1 -> Mux1/5
  I D/1 -> Mux1/4
  U E/1 -> Mux/5
  U D/1 -> Mux/4
  I C:/1 -> Mux1/3
  I B:/1 -> Mux1/2
  I A:/1 -> Mux1/1
  Mux1/1 -> i/1
  Mux/1 -> v/1
  U C:/1 -> Mux/3
  U B:/1 -> Mux/2
  U A:/1 -> Mux/1
  connections:
  I E/RConn1 -- e/RConn1
  I D/RConn1 -- d/RConn1
  U E/LConn1 -- Multimeter4/LConn1 -- I E/LConn1 -- E/RConn1
  U D/LConn1 -- Multimeter3/LConn1 -- I D/LConn1 -- D/RConn1
  U E/LConn2 -- U D/LConn2 -- U A:/LConn2 -- U B:/LConn2 -- U C:/LConn2 -- Ground/LConn1
  I C:/RConn1 -- c/RConn1
  U B:/LConn1 -- B/RConn1 -- Multimeter1/LConn1 -- I B:/LConn1
  U C:/LConn1 -- C/RConn1 -- Multimeter2/LConn1 -- I C:/LConn1
  a/RConn1 -- I A:/RConn1
  I B:/RConn1 -- b/RConn1
  U A:/LConn1 -- A/RConn1 -- Multimeter/LConn1 -- I A:/LConn1
